simulink model "hdl_learn_counter"  (R2025b)
settings: Solver=FixedStepDiscrete  StartTime=0.0  StopTime=20  RelTol=1e-3
settings Model: DataTypeOverride=Off  Creator=kimsteph  LastModifiedBy=kimsteph
settings OptimizationCC: BlockReduction=off  ConditionallyExecuteInputs=off  DefaultParameterBehavior=Inlined  InheritOutputTypeSmallerThanSingle=on
settings DebuggingCC: ArtificialAlgebraicLoopMsg=error  SingleTaskRateTransMsg=error
settings HardwareCC: ProdBitPerPointer=32.0  ProdBitPerSizeT=32.0  ProdBitPerPtrDiffT=32.0  ProdLargestAtomicFloat=None  ProdIntDivRoundTo=Undefined  ProdEndianess=Unspecified  ProdWordSize=32.0  ProdHWDeviceType=ASIC/FPGA->ASIC/FPGA  TargetBitPerPointer=64.0  TargetBitPerSizeT=64.0  TargetBitPerPtrDiffT=64.0  TargetLongLongMode=on  TargetIntDivRoundTo=Zero  TargetEndianess=LittleEndian  TargetWordSize=64.0  TargetHWDeviceType=Custom Processor->MATLAB Host Computer  ProdEqTarget=off

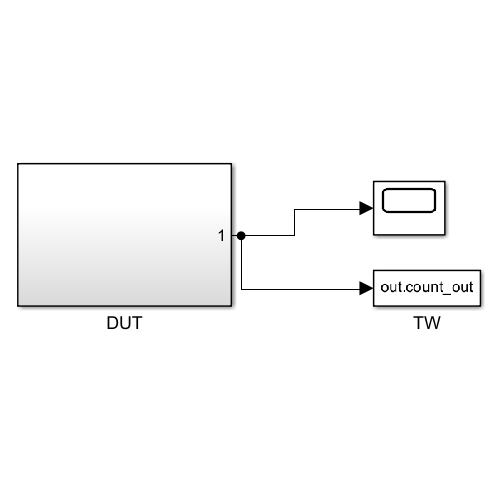
[thumbnail: Simulink's stored preview of the top-level diagram]
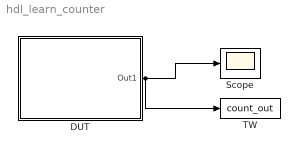
== system hdl_learn_counter ==
  DUT : Subsystem
  Scope : Scope
  TW : ToWorkspace  VariableName=count_out  SaveFormat=Timeseries  SampleTime=-1
  wires:
  DUT/1(Out1) -> Scope/1, TW/1

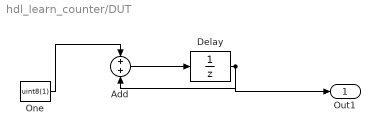
== system hdl_learn_counter/DUT ==
  Add : Sum  OutDataTypeStr=uint8  SaturateOnIntegerOverflow=on
  Delay : UnitDelay  HasFrameUpgradeWarning=on
  One : Constant  Value=uint8(1)  OutDataTypeStr=uint8
  Out1 : Outport
  wires:
  One/1 -> Add/1
  Delay/1 -> Add/2, Out1/1
  Add/1 -> Delay/1
